simulink model "sf_aircontrol"  (Simulink 7.6)
settings: Solver=ode45  StartTime=0.0  StopTime=600  FixedStep=1000  RelTol=1e-3
undefined symbols (not defined in the file or in its folder): sigbuilder_block
settings Model: Creator=The MathWorks Inc.  ExtModeAutoUpdateStatusClock=off
settings SolverCC: MaxConsecutiveZCs=500
settings OptimizationCC: InitFltsAndDblsToZero=on
settings DebuggingCC: SaveWithParameterizedLinksMsg=none  SignalResolutionControl=TryResolveAllWithWarning  SolverPrmCheckMsg=none  MultiTaskDSMMsg=warning  MultiTaskCondExecSysMsg=none  StrictBusMsg=Warning
settings SFSimCC: SimParseCustomCode=off
settings RTWCC: IncludeERTFirstTime=on
settings CodeAppCC: CustomSymbolStrFcn=$F$N$M
settings GRTTargetCC: TargetFcnLib=ansi_tfl_tmw.mat

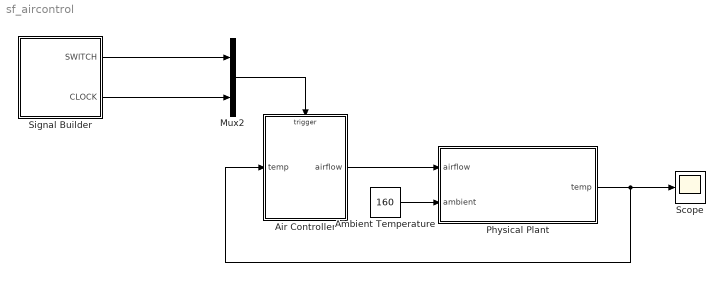
== system sf_aircontrol ==
  Air Controller : Stateflow chart  TreatAsAtomicUnit=on
  Ambient Temperature : Constant  Value=160
  Mux2 : Mux  Inputs=2
  Physical Plant : Subsystem
  Scope : Scope
      settings: TimeRange=600  YMin=60  YMax=160
  Signal Builder : Subsystem  Tag=STV Subsys  LoadFcn=sigbuilder_block('load');  StartFcn=sigbuilder_block('start');  StopFcn=sigbuilder_block('stop');  ClipboardFcn=sigbuilder_block('clipboard');  mask(Sigbuilder block){}
      mask help: Sigbuilder GUI
      mask init:
      | if ~strcmp(get_param(bdroot(gcbh),'SimulationStatus'),'stopped') tuvar = sigbuilder_block('maskInit'); end
      settings: CopyFcn=sigbuilder_block('copy');  DeleteFcn=sigbuilder_block('delete');  ModelCloseFcn=sigbuilder_block('modelClose');  PreSaveFcn=sigbuilder_block('preSave');  NameChangeFcn=sigbuilder_block('namechange');  OpenFcn=sigbuilder_block('open',[88.3417 74.8984 604.949 351.446 ]);  CloseFcn=sigbuilder_block('close');
      mask Display: plot(0,0,100,100,[10,10,40,40,10],[80,20,20,80,80],[40,10],[50,50], [40,27,10],[65,72,56],[40,25,25,10],[28,28,43,43]);
  wires:
  Mux2/1 -> Air Controller/Trigger
  Air Controller/1(airflow) -> Physical Plant/1(airflow)
  Ambient Temperature/1 -> Physical Plant/2(ambient)
  Physical Plant/1(temp) -> Scope/1, Air Controller/1(temp)
  Signal Builder/1(SWITCH) -> Mux2/1
  Signal Builder/2(CLOCK) -> Mux2/2

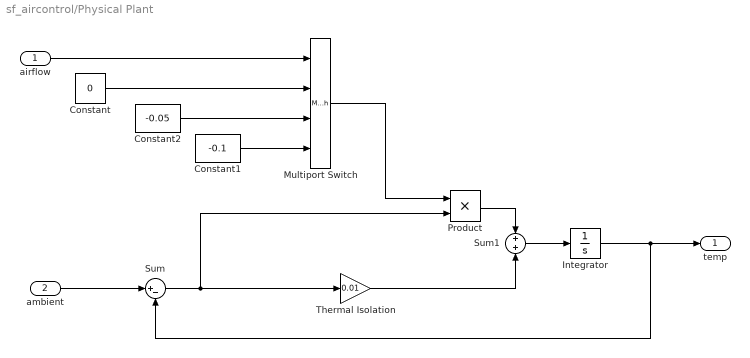
== system sf_aircontrol/Physical Plant ==
  airflow : Inport
  ambient : Inport  Port=2
  Constant : Constant  Value=0
  Constant1 : Constant  Value=-0.1
  Constant2 : Constant  Value=-0.05
  Integrator : Integrator  InitialCondition=70
  Multiport Switch : MultiPortSwitch  DataPortOrder=Zero-based contiguous  zeroidx=on
  Product : Product  RndMeth=Zero
  Sum : Sum  Inputs=|+-
  Sum1 : Sum  Inputs=+|+
  Thermal Isolation : Gain  Gain=0.01
  temp : Outport
  wires:
  Integrator/1 -> temp/1, Sum/2
  Sum1/1 -> Integrator/1
  Constant2/1 -> Multiport Switch/3
  Constant/1 -> Multiport Switch/2
  airflow/1 -> Multiport Switch/1
  ambient/1 -> Sum/1
  Sum/1 -> Thermal Isolation/1, Product/2
  Product/1 -> Sum1/1
  Thermal Isolation/1 -> Sum1/2
  Multiport Switch/1 -> Product/1
  Constant1/1 -> Multiport Switch/4

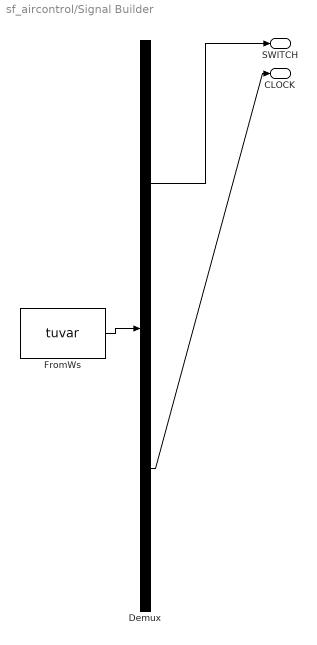
== system sf_aircontrol/Signal Builder ==
  Demux : Demux  Tag=STV Demux  Outputs=2
  FromWs : FromWorkspace  Tag=STV FromWs  VariableName=tuvar  SampleTime=0  SigBuilderData=DataTag0  VnvData=DataTag1
      SigBuilderData=|
      | common.afterFinalStr = 'Extrapolate'
      | common.sampleTime = 0
      | dataSet.timeRange = [0 600]
      | dataSet.name = 'Group 1'
      | sbobj.Groups.Name = 'Group 1'
      | sbobj.Groups.Signals(1).Name = 'SWITCH'
      | sbobj.Groups.Signals(1).XData = [0 350 350 501 501 600]
      | sbobj.Groups.Signals(1).YData = [0 -0.01 1 1 0 0]
      | sbobj.Groups.Signals(2).Name = 'CLOCK'
      | sbobj.Groups.Signals(2).XData = [0 0.5 0.5 1 1 1.5 1.5 2 2 2.5 2.5 3 ... (2397 elements, 1x2397)]
      | sbobj.Groups.Signals(2).YData = [2 2 0 0 2 2 0 0 2 2 0 0 ... (2397 elements, 1x2397)]
      | sbobj.Groups.TimeRange = [0 600]
  SWITCH : Outport  Tag=STV Outport
  CLOCK : Outport  Tag=STV Outport  Port=2
  wires:
  Demux/1 -> SWITCH/1
  FromWs/1 -> Demux/1
  Demux/2 -> CLOCK/1

== stateflow chart Air Controller ==
  state PowerOn
    state FAN2 [parallel]
      settings: executionOrder=2
      state Off
      state On
      PowerOn.FAN2.On -> PowerOn.FAN2.Off : [temp<150]
      PowerOn.FAN2.Off -> PowerOn.FAN2.On : [temp>=150]
      (default) -> PowerOn.FAN2.Off
    state SpeedValue [parallel]
      du: airflow = in(FAN1.On) + in(FAN2.On);
      settings: executionOrder=3
    state FAN1 [parallel]
      settings: executionOrder=1
      state Off
      state On
      (default) -> PowerOn.FAN1.Off
      PowerOn.FAN1.Off -> PowerOn.FAN1.On : [temp >=120]
      PowerOn.FAN1.On -> PowerOn.FAN1.Off : [temp < 120]
  state PowerOff
    en:
    airflow = 0;
  (default) -> PowerOff
  PowerOff -> PowerOn : SWITCH
  PowerOn -> PowerOff : SWITCH
  data: airflow output uint8; temp input double
  events: SWITCH input EITHER_EDGE_EVENT; CLOCK input EITHER_EDGE_EVENT
